simulink model "Lab1P2Si"  (R2021a)
settings: Solver=VariableStepAuto  StartTime=0.0  StopTime=15.0  MaxStep=0.0001  RelTol=1e-3
settings Model: Creator=kkqi_  LastModifiedBy=afayeed

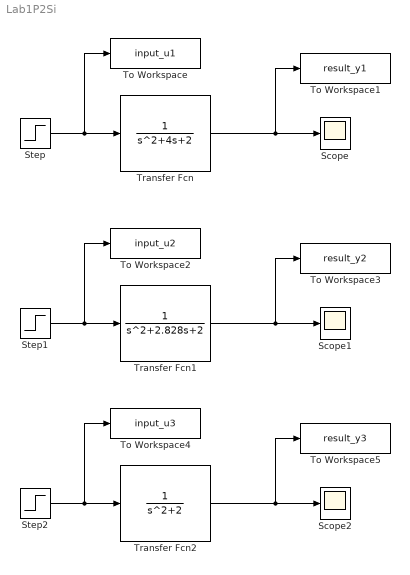
== system Lab1P2Si ==
  Scope : Scope
  Scope1 : Scope
  Scope2 : Scope
  Step : Step  Time=0  SampleTime=0
  Step1 : Step  Time=0  SampleTime=0
  Step2 : Step  Time=0  SampleTime=0
  To Workspace : ToWorkspace  VariableName=input_u1  SampleTime=-1
  To Workspace1 : ToWorkspace  VariableName=result_y1  SampleTime=-1
  To Workspace2 : ToWorkspace  VariableName=input_u2  SampleTime=-1
  To Workspace3 : ToWorkspace  VariableName=result_y2  SampleTime=-1
  To Workspace4 : ToWorkspace  VariableName=input_u3  SampleTime=-1
  To Workspace5 : ToWorkspace  VariableName=result_y3  SampleTime=-1
  Transfer Fcn : TransferFcn  Denominator=[1 4 2]
  Transfer Fcn1 : TransferFcn  Denominator=[1 2.828 2]
  Transfer Fcn2 : TransferFcn  Denominator=[1 0 2]
  wires:
  Step/1 -> To Workspace/1, Transfer Fcn/1
  Transfer Fcn/1 -> To Workspace1/1, Scope/1
  Step1/1 -> To Workspace2/1, Transfer Fcn1/1
  Transfer Fcn1/1 -> To Workspace3/1, Scope1/1
  Transfer Fcn2/1 -> To Workspace5/1, Scope2/1
  Step2/1 -> To Workspace4/1, Transfer Fcn2/1
